simulink model "Test_motors"  (R2022a)
settings: Solver=VariableStepAuto  StartTime=0.0  StopTime=10  RelTol=1e-3
values from neighbouring files (symbols this model uses):
  Ia_init = 0    [ELEN90064_Project_Parameters.m]    (also in mpc_example_regulation.m; mpc_example_tracking.m)
libraries: simulink x1
settings Model: Creator=Admin  LastModifiedBy=Admin

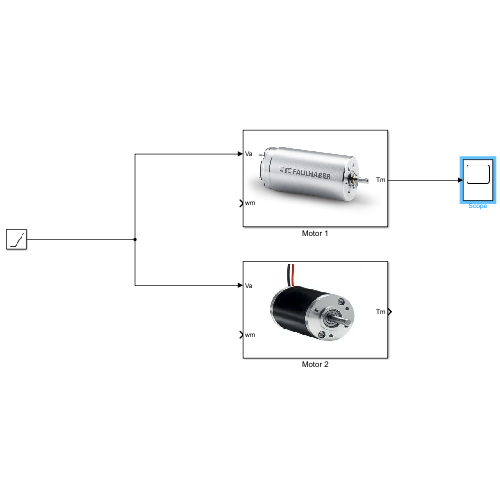
[thumbnail: Simulink's stored preview of the top-level diagram]
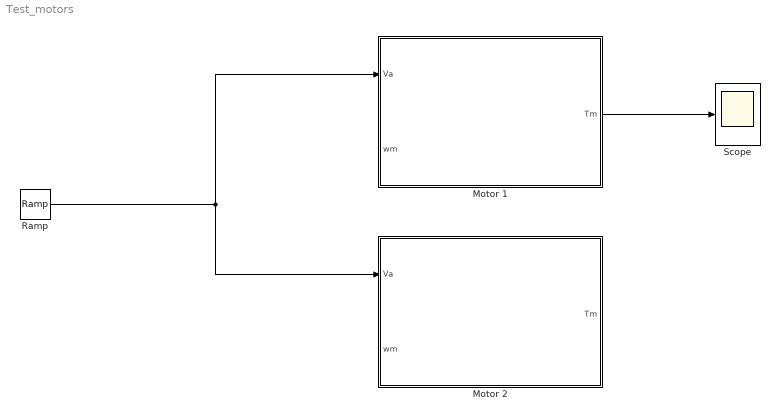
== system Test_motors ==
  Motor 1 : Subsystem
      mask Display: image('$imagefile'); % Use "Edit Image" on toolstrip to change.
  Motor 2 : Subsystem
      mask Display: image('$imagefile'); % Use "Edit Image" on toolstrip to change.
  Ramp : simulink/Sources/Ramp  slope=1  start=0  InitialOutput=0
  Scope : Scope
  wires:
  Ramp/1 -> Motor 1/1(Va), Motor 2/1(Va)
  Motor 1/1(Tm) -> Scope/1

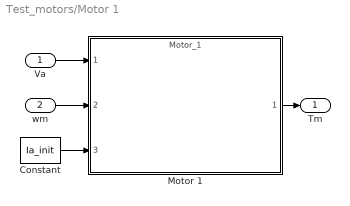
== system Test_motors/Motor 1 ==
  Va : Inport
  wm : Inport  Port=2
  Constant : Constant  Value=Ia_init
  Motor 1 : ModelReference  ModelNameDialog=Motor_1  ModelReferenceVersion=1.18  CopyOfModelProtected=on
  Tm : Outport
  wires:
  Constant/1 -> Motor 1/3
  Motor 1/1 -> Tm/1
  wm/1 -> Motor 1/2
  Va/1 -> Motor 1/1

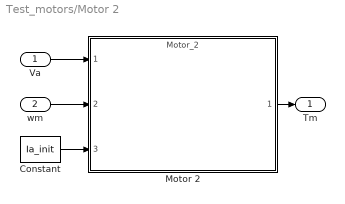
== system Test_motors/Motor 2 ==
  Va : Inport
  wm : Inport  Port=2
  Constant : Constant  Value=Ia_init
  Motor 2 : ModelReference  ModelNameDialog=Motor_2  ModelReferenceVersion=1.19  CopyOfModelProtected=on
  Tm : Outport
  wires:
  Constant/1 -> Motor 2/3
  wm/1 -> Motor 2/2
  Va/1 -> Motor 2/1
  Motor 2/1 -> Tm/1
